simulink model "InversePendulum"  (R2023b)
settings: Solver=VariableStepAuto  StartTime=0.0  StopTime=15
model workspace: external: MAT-File ./params.mat (data not in the file)
values from neighbouring files (symbols this model uses):
  force_limits = [-100 100]    [params.mat]
  grav = 9.81    [params.mat]
  K = [-100 -159.964433227 -823.481805968 -207.917391727]    [params.mat]
  len = 0.5    [params.mat]
  mass = 1    [params.mat]
  mass_cart = 5    [params.mat]
  x_init = [0 0 0.785398163397 0]    [params.mat]
settings Model: Creator=anigo  LastModifiedBy=ishan
settings OptimizationCC: ReuseModelBlockBuffer=off

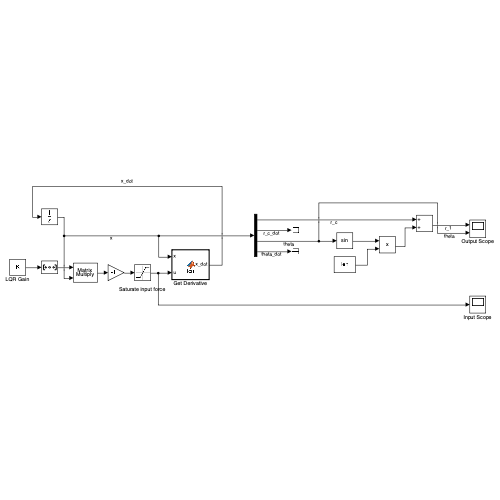
[thumbnail: Simulink's stored preview of the top-level diagram]
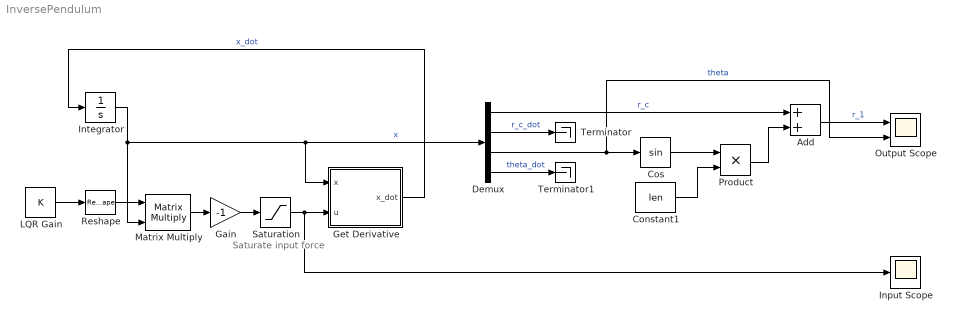
== system InversePendulum ==
  note: Saturate input force
  Add : Sum
  Constant1 : Constant  Value=len
  Cos : Trigonometry
  Demux : Demux
  Gain : Gain  Gain=-1
  Get Derivative : MATLAB Function  TreatAsAtomicUnit=on
  Input Scope : Scope
  Integrator : Integrator  InitialCondition=x_init
  LQR Gain : Constant  Value=K  OutDataTypeStr=Inherit: Inherit via back propagation
  Matrix Multiply : Product  Multiplication=Matrix(*)
  Output Scope : Scope  NumInputPorts=2
  Product : Product
  Reshape : Reshape  OutputDimensionality=Row vector (2-D)
  Saturation : Saturate  UpperLimit=force_limits(2)  LowerLimit=force_limits(1)
  Terminator : Terminator
  Terminator1 : Terminator
  wires:
  Get Derivative/1(x_dot) -> Integrator/1  "x_dot"
  Integrator/1 -> Get Derivative/1(x), Demux/1, Matrix Multiply/2  "x"
  Matrix Multiply/1 -> Gain/1
  Demux/1 -> Add/1  "r_c"
  Demux/2 -> Terminator/1  "r_c_dot"
  Demux/3 -> Output Scope/2, Cos/1  "theta"
  Demux/4 -> Terminator1/1  "theta_dot"
  Product/1 -> Add/2
  Cos/1 -> Product/1
  Constant1/1 -> Product/2
  Add/1 -> Output Scope/1  "r_1"
  LQR Gain/1 -> Reshape/1
  Reshape/1 -> Matrix Multiply/1
  Gain/1 -> Saturation/1
  Saturation/1 -> Input Scope/1, Get Derivative/2(u)

== matlab function InversePendulum/Get Derivative ==
  data: x input; x_dot output; u input; grav parameter; mass parameter; mass_cart parameter; len parameter
function x_dot = fcn(x, u, grav, mass, mass_cart, len)
r_dot_c = x(2);
theta = x(3);
theta_dot = x(4);

x_dot = [r_dot_c; (u*sin(theta) - grav*mass*cos(theta) + u*cos(theta)*cot(theta) + len*mass*theta_dot^2*cos(theta)^2 + len*mass*theta_dot^2*sin(theta)^2)/(mass*sin(theta) + mass_cart*sin(theta) + mass_cart*cos(theta)*cot(theta)); theta_dot; (grav*mass + grav*mass_cart - u*cot(theta) - len*mass*theta_dot^2*cos(theta) - len*mass_cart*theta_dot^2*cos(theta) + len*mass_cart*theta_dot^2*cot(theta)*sin(theta))/(len*(mass*sin(theta) + mass_cart*sin(theta) + mass_cart*cos(theta)*cot(theta)))];
